simulink model "rezervoarjednacine"  (R2012b)
settings: Solver=ode45  StartTime=0.0  StopTime=10.0  RelTol=1e-3
settings Model: Creator=korisnik  LastModifiedBy=korisnik

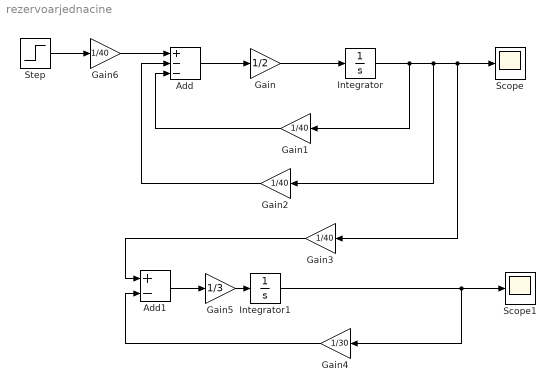
== system rezervoarjednacine ==
  Add : Sum  Inputs=+--
  Add1 : Sum  Inputs=+-
  Gain : Gain  Gain=1/2
  Gain{1..3,6} (4 alike) : Gain  Gain=1/40
  Gain4 : Gain  Gain=1/30
  Gain5 : Gain  Gain=1/3
  Integrator : Integrator
  Integrator1 : Integrator
  Scope : Scope
  Scope1 : Scope
  Step : Step  Time=0  SampleTime=0
  wires:
  Gain/1 -> Integrator/1
  Integrator/1 -> Gain1/1, Gain2/1, Gain3/1, Scope/1
  Add/1 -> Gain/1
  Gain1/1 -> Add/3
  Gain2/1 -> Add/2
  Gain3/1 -> Add1/1
  Add1/1 -> Gain5/1
  Integrator1/1 -> Gain4/1, Scope1/1
  Gain4/1 -> Add1/2
  Gain5/1 -> Integrator1/1
  Step/1 -> Gain6/1
  Gain6/1 -> Add/1
